simulink model "integral_control"  (R2024b)
settings: Solver=VariableStepAuto  StartTime=0.0  StopTime=20  RelTol=1e-3
values from neighbouring files (symbols this model uses):
  A = output{1}    [task5.m]
  B = output{2}    [task5.m]
  C = output{3}    [task5.m]
  K = R\B_bar'*P    [task5.m]
  L = K_tilde'    [task5.m]
  w = [-1;1]    [task5.m]
  y_sp = output{4}    [task5.m]
settings Model: Creator=wyton  LastModifiedBy=KevinNuo
settings SolverCC: AlgebraicLoopSolver=TrustRegion
settings OptimizationCC: ReuseModelBlockBuffer=off
settings DebuggingCC: UnconnectedInputMsg=warning  UnconnectedOutputMsg=warning  UnconnectedLineMsg=warning
settings ModelReferenceCC: EnableRefExpFcnMdlSchedulingChecks=on
settings RTWCC: GPUComputeCapability=3.5  DLArmComputeVersion=19.05

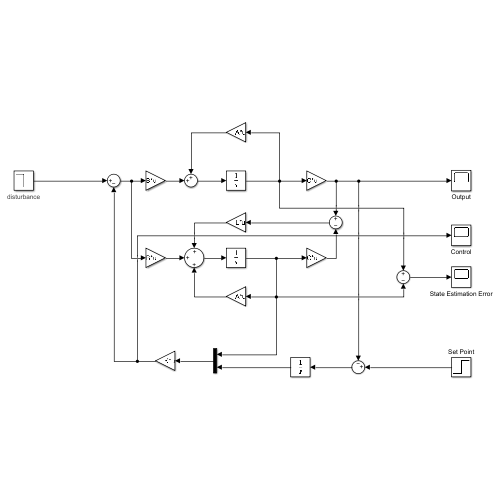
[thumbnail: Simulink's stored preview of the top-level diagram]
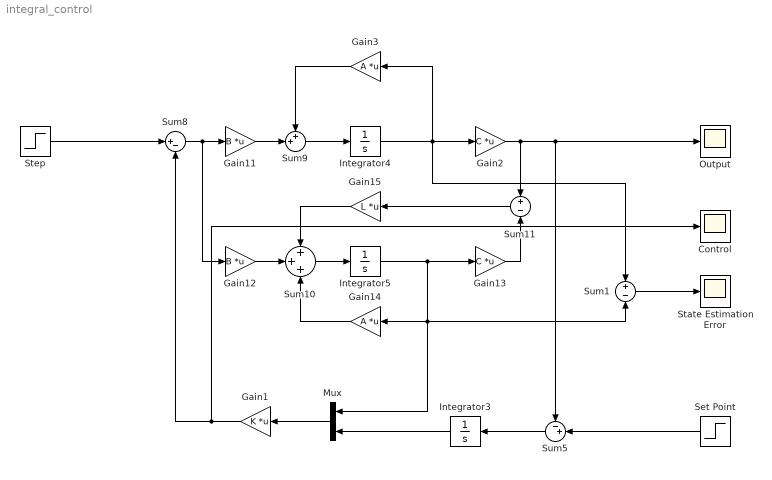
== system integral_control ==
  Control : Scope
  Gain1 : Gain  Gain=K  Multiplication=Matrix(K*u)
  Gain11 : Gain  Gain=B  Multiplication=Matrix(K*u)
  Gain12 : Gain  Gain=B  Multiplication=Matrix(K*u)
  Gain13 : Gain  Gain=C  Multiplication=Matrix(K*u)
  Gain14 : Gain  Gain=A  Multiplication=Matrix(K*u)
  Gain15 : Gain  Gain=L  Multiplication=Matrix(K*u)
  Gain2 : Gain  Gain=C  Multiplication=Matrix(K*u)
  Gain3 : Gain  Gain=A  Multiplication=Matrix(K*u)
  Integrator3 : Integrator
  Integrator4 : Integrator
  Integrator5 : Integrator
  Mux : Mux  Inputs=2
  Output : Scope
  Set Point : Step  Time=0  Before=[0;0;0]  After=y_sp  SampleTime=0
  State Estimation Error : Scope
  Step : Step  Time=10  Before=[0;0]  After=w  SampleTime=0
      settings: AttributesFormatString=disturbance
  Sum1 : Sum  Inputs=+|-
  Sum10 : Sum  Inputs=+++
  Sum11 : Sum  Inputs=+|-
  Sum5 : Sum  Inputs=-+|
  Sum8 : Sum  Inputs=|+-
  Sum9 : Sum  Inputs=++|
  wires:
  Gain14/1 -> Sum10/3
  Gain2/1 -> Sum11/1, Output/1, Sum5/1
  Integrator4/1 -> Gain3/1, Gain2/1, Sum1/1
  Gain13/1 -> Sum11/2
  Sum8/1 -> Gain12/1, Gain11/1
  Gain11/1 -> Sum9/2
  Gain3/1 -> Sum9/1
  Sum9/1 -> Integrator4/1
  Gain12/1 -> Sum10/2
  Sum11/1 -> Gain15/1
  Integrator3/1 -> Mux/2
  Gain15/1 -> Sum10/1
  Integrator5/1 -> Sum1/2, Mux/1, Gain14/1, Gain13/1
  Sum5/1 -> Integrator3/1
  Sum10/1 -> Integrator5/1
  Step/1 -> Sum8/1
  Set Point/1 -> Sum5/2
  Mux/1 -> Gain1/1
  Gain1/1 -> Control/1, Sum8/2
  Sum1/1 -> State Estimation Error/1
